simulink model "rlDDPGmdl"  (R2021a)
settings: Solver=VariableStepAuto  StartTime=0.0  StopTime=10.0  RelTol=1e-3
model workspace (MAT data in the model file):
  I = 0
  Sig = Simulink.Signal
  Sig.DataType = 'auto'
  Sig.Dimensions = -1
  Sig.DimensionsMode = 'auto'
  Sig.Complexity = 'auto'
  Sig.SampleTime = -1
  Sig.SamplingMode = 'auto'
  Sig1 = Simulink.Signal
  Sig1.DataType = 'auto'
  Sig1.Dimensions = -1
  Sig1.DimensionsMode = 'auto'
  Sig1.Complexity = 'auto'
  Sig1.SampleTime = -1
  Sig1.SamplingMode = 'auto'
  c = 0
  g = 10
  g_original = 9.81
  l = 1
  m = 1
  max_tau = 15
  max_tau_original = 2
  theta0 = 0
  theta_dot0 = 0
libraries: rllib x1
settings Model: OrderedModelArguments=off  Creator=wogwan  LastModifiedBy=wogwan

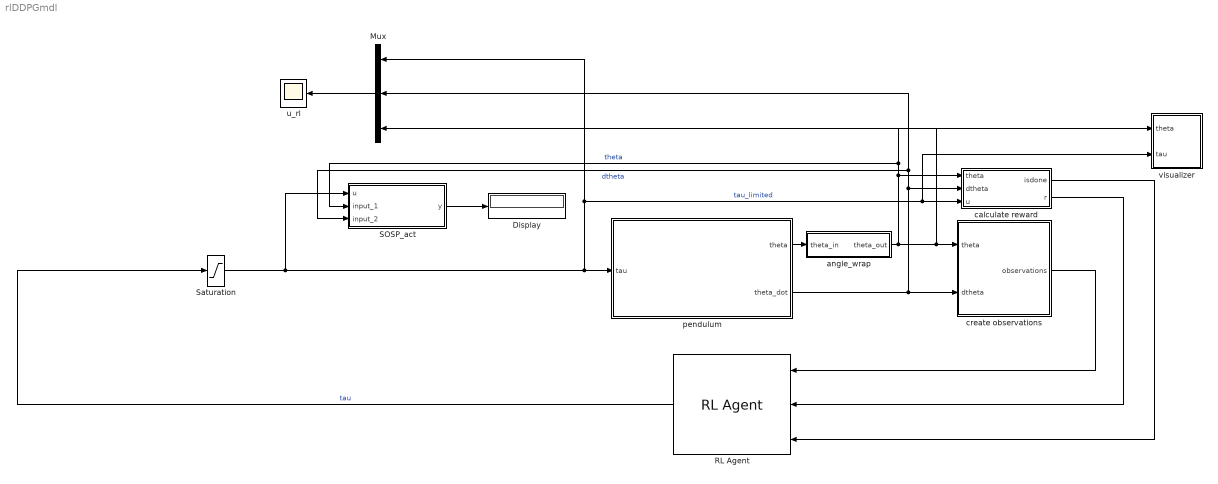
== system rlDDPGmdl ==
  Display : Display
  Mux : Mux  Inputs=3
  RL Agent : rllib/RL Agent  Agent=agent  ExternalActionAsInput=off  ProvideCumRwd=off  TreatAsDirectFeedthrough=on
  SOSP_act : MATLAB Function  TreatAsAtomicUnit=on
  Saturation : Saturate  UpperLimit=max_tau  LowerLimit=-max_tau
  angle_wrap : Subsystem
  calculate reward : Subsystem
  create observations : Subsystem  Variant=on  VariantControlMode=label  VariantControl=Variant1  LabelModeActiveChoice=sincos  mask{ThetaObservationHandling=sincos}
      mask prompts: ThetaObservationHandling "Select how theta is treated in the observation vector"
      mask init:
      | simulationStatus = get_param(bdroot,'SimulationStatus');
      | 
      | % The active variant can only be modified at edit-time or very early during
      | % the simulink compile stage. 
      | 
      | choice = get_param(gcb,'ThetaObservationHandling');
      | oldVariant = get_param(gcb,'OverrideUsingVariant');
      | 
      | switch choice
      |     case 'theta'
      |     case 'sincos'
      |     otherwise
      |         error('%s is not supported',choice)
      | end
      | set_param(gcb,'OverrideUsingVariant',choice);
      mask TypeOptions ThetaObservationHandling: theta | sincos
  pendulum : Subsystem
  u_rl : Scope
  visualizer : Subsystem
  wires:
  create observations/1(" observations") -> RL Agent/1
  angle_wrap/1(theta_out) -> SOSP_act/2(input_1), visualizer/1(theta), calculate reward/1(theta), Mux/3, create observations/1("theta ")  "theta"
  calculate reward/1(isdone) -> RL Agent/3
  Saturation/1 -> Mux/1, visualizer/2(tau), calculate reward/3(u), pendulum/1(tau), SOSP_act/1(u)  "tau_limited"
  RL Agent/1 -> Saturation/1  "tau"
  calculate reward/2(r) -> RL Agent/2
  pendulum/1(theta) -> angle_wrap/1(theta_in)
  pendulum/2(theta_dot) -> SOSP_act/3(input_2), Mux/2, calculate reward/2(dtheta), create observations/2("dtheta ")  "dtheta"
  Mux/1 -> u_rl/1
  SOSP_act/1(y) -> Display/1

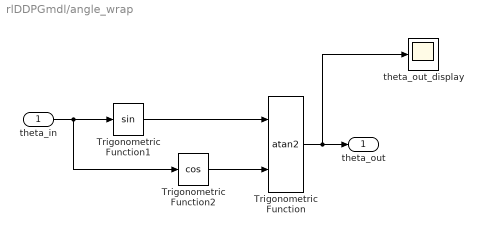
== system rlDDPGmdl/angle_wrap ==
  theta_in : Inport
  Trigonometric Function : Trigonometry  Operator=atan2
  Trigonometric Function1 : Trigonometry
  Trigonometric Function2 : Trigonometry  Operator=cos
  theta_out_display : Scope
  theta_out : Outport  VectorParamsAs1DForOutWhenUnconnected=off
  wires:
  theta_in/1 -> Trigonometric Function2/1, Trigonometric Function1/1
  Trigonometric Function/1 -> theta_out_display/1, theta_out/1
  Trigonometric Function1/1 -> Trigonometric Function/1
  Trigonometric Function2/1 -> Trigonometric Function/2

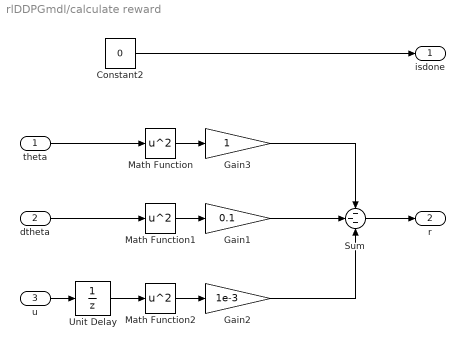
== system rlDDPGmdl/calculate reward ==
  theta : Inport
  dtheta : Inport  Port=2
  u : Inport  Port=3
  Constant2 : Constant  Value=0
  Gain1 : Gain  Gain=0.1
  Gain2 : Gain  Gain=1e-3
  Gain3 : Gain
  Math Function : Math  Operator=square  SignedPower=on  SaturateOnIntegerOverflow=on
  Math Function1 : Math  Operator=square  SignedPower=on  SaturateOnIntegerOverflow=on
  Math Function2 : Math  Operator=square  SignedPower=on  SaturateOnIntegerOverflow=on
  Sum : Sum  Inputs=---
  Unit Delay : UnitDelay  SampleTime=-1  HasFrameUpgradeWarning=on
  isdone : Outport  VectorParamsAs1DForOutWhenUnconnected=off
  r : Outport  Port=2  VectorParamsAs1DForOutWhenUnconnected=off
  wires:
  Constant2/1 -> isdone/1
  theta/1 -> Math Function/1
  dtheta/1 -> Math Function1/1
  u/1 -> Unit Delay/1
  Sum/1 -> r/1
  Math Function/1 -> Gain3/1
  Math Function1/1 -> Gain1/1
  Math Function2/1 -> Gain2/1
  Gain2/1 -> Sum/3
  Gain1/1 -> Sum/2
  Gain3/1 -> Sum/1
  Unit Delay/1 -> Math Function2/1

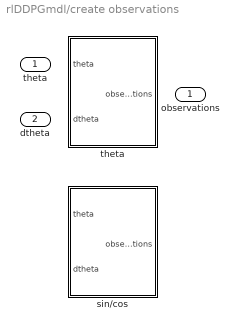
== system rlDDPGmdl/create observations ==
  "theta " : Inport
  "dtheta " : Inport  Port=2
  sin/cos : Subsystem  VariantControl=sincos
  theta : Subsystem  VariantControl=theta
  " observations" : Outport  VectorParamsAs1DForOutWhenUnconnected=off

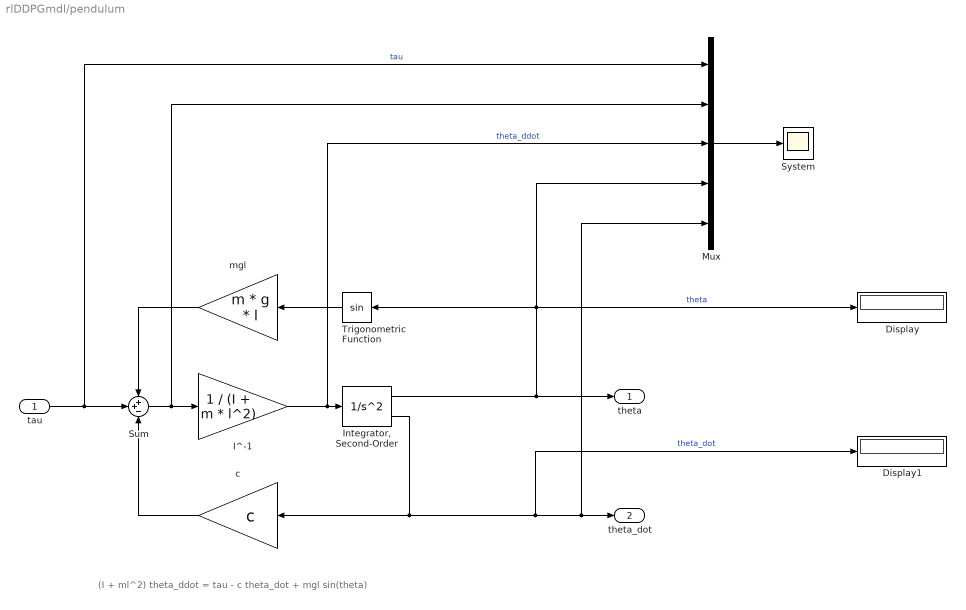
== system rlDDPGmdl/pendulum ==
  note: (I + ml^2) theta_ddot = tau - c theta_dot + mgl sin(theta)
  tau : Inport
  Display : Display
  Display1 : Display
  I^-1 : Gain  Gain=1 / (I + m * l^2)
  "Integrator, Second-Order" : SecondOrderIntegrator  ICX=theta0  UpperLimitX=1  LowerLimitX=0  StateNameX='theta'  ICDXDT=theta_dot0  StateNameDXDT='theta_dot'
  Mux : Mux  Inputs=5
  Sum : Sum  Inputs=++-
  System : Scope
  Trigonometric Function : Trigonometry
  c : Gain  Gain=c
  mgl : Gain  Gain=m * g * l
  theta : Outport  VectorParamsAs1DForOutWhenUnconnected=off
  theta_dot : Outport  Port=2  VectorParamsAs1DForOutWhenUnconnected=off
  wires:
  mgl/1 -> Sum/1
  c/1 -> Sum/3
  Trigonometric Function/1 -> mgl/1
  Sum/1 -> Mux/2, I^-1/1
  "Integrator, Second-Order"/1 -> Display/1, Trigonometric Function/1, Mux/4, theta/1  "theta"
  I^-1/1 -> Mux/3, "Integrator, Second-Order"/1  "theta_ddot"
  "Integrator, Second-Order"/2 -> c/1, Display1/1, Mux/5, theta_dot/1  "theta_dot"
  tau/1 -> Sum/2, Mux/1  "tau"
  Mux/1 -> System/1

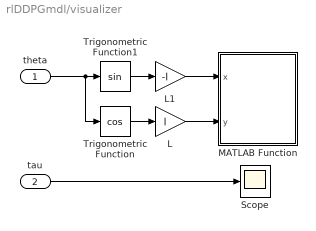
== system rlDDPGmdl/visualizer ==
  theta : Inport
  tau : Inport  Port=2
  L : Gain  Gain=l
  L1 : Gain  Gain=-l
  MATLAB Function : MATLAB Function  TreatAsAtomicUnit=on
  Scope : Scope
  Trigonometric Function : Trigonometry  Operator=cos
  Trigonometric Function1 : Trigonometry
  wires:
  theta/1 -> Trigonometric Function/1, Trigonometric Function1/1
  L1/1 -> MATLAB Function/1(x)
  Trigonometric Function/1 -> L/1
  L/1 -> MATLAB Function/2(y)
  Trigonometric Function1/1 -> L1/1
  tau/1 -> Scope/1

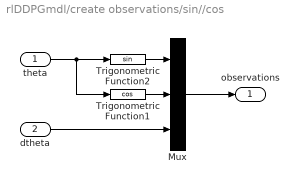
== system rlDDPGmdl/create observations/sin//cos ==
  theta : Inport
  dtheta : Inport  Port=2
  Mux : Mux  Inputs=3
  Trigonometric Function1 : Trigonometry  Operator=cos
  Trigonometric Function2 : Trigonometry
  observations : Outport  VectorParamsAs1DForOutWhenUnconnected=off
  wires:
  theta/1 -> Trigonometric Function1/1, Trigonometric Function2/1
  Mux/1 -> observations/1
  dtheta/1 -> Mux/3
  Trigonometric Function2/1 -> Mux/1
  Trigonometric Function1/1 -> Mux/2

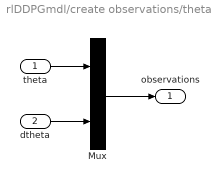
== system rlDDPGmdl/create observations/theta ==
  theta : Inport
  dtheta : Inport  Port=2
  Mux : Mux  Inputs=2
  observations : Outport  VectorParamsAs1DForOutWhenUnconnected=off
  wires:
  dtheta/1 -> Mux/2
  Mux/1 -> observations/1
  theta/1 -> Mux/1

== matlab function rlDDPGmdl/SOSP_act ==
  data: u input; y output; input_1 input; input_2 input
function y = fcn(u, input_1, input_2)
coder.extrinsic('sys_compute');
y = 0;
y = sos_compute(u,input_1,input_2);
end

== matlab function rlDDPGmdl/visualizer/MATLAB Function ==
  settings: updateMethod=DISCRETE
  data: x input; y input
function plotPend(x,y)
% plot the simple pendulum
coder.extrinsic('rl.env.viz.plotSimplePendulum');
rl.env.viz.plotSimplePendulum(x,y);
